simulink model "ThermalConv"  (R2023b)
settings: Solver=FixedStepDiscrete  StartTime=0.0  StopTime=10.0  FixedStep=10e-3  RelTol=1e-3
libraries: AswLib x12
settings Model: DataDictionary=ThermalConv.sldd  Creator=84339  LastModifiedBy=84339
settings OptimizationCC: DefaultParameterBehavior=Inlined  EnhancedBackFolding=on  PassReuseOutputArgsAs=Individual arguments  ZeroExternalMemoryAtStartup=off  ZeroInternalMemoryAtStartup=off  OptimizeBlockOrder=speed  DifferentSizesBufferReuse=on  OptimizationCustomize=off  EfficientTunableParamExpr=on
settings DebuggingCC: ParameterTunabilityLossMsg=error
settings SFSimCC: MATLABDynamicMemAlloc=off
settings RTWCC: Description=Embedded Coder  SystemTargetFile=ert.tlc  EmbeddedCoderDictionary=ASW.sldd  GenCodeOnly=on  TemplateMakefile=ert_default_tmf  DataTypeReplacement=CDataTypesFixedWidth
settings CodeAppCC: ForceParamTrailComments=on  IgnoreCustomStorageClasses=off  OperatorAnnotations=on  SimulinkDataObjDesc=on  SFDataObjDesc=on  InsertBlockDesc=on
settings ERTTargetCC: TargetLangStandard=C99 (ISO)  GenerateSampleERTMain=on  InlinedParameterPlacement=NonHierarchical  ERTCustomFileTemplate=example_file_process.tlc  MaxIdInt64=INT64_MAX  MinIdInt64=INT64_MIN  MaxIdUint64=UINT64_MAX  MaxIdInt32=INT32_MAX  MinIdInt32=INT32_MIN  MaxIdUint32=UINT32_MAX  MaxIdInt16=INT16_MAX  MinIdInt16=INT16_MIN  MaxIdUint16=UINT16_MAX  MaxIdInt8=INT8_MAX  MinIdInt8=INT8_MIN  MaxIdUint8=UINT8_MAX

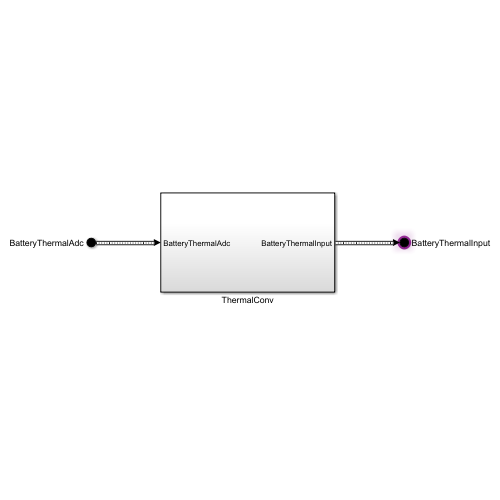
[thumbnail: Simulink's stored preview of the top-level diagram]
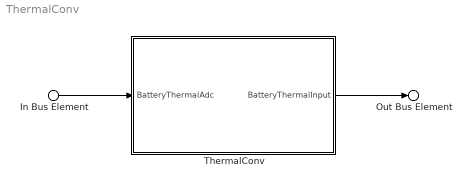
== system ThermalConv ==
  In Bus Element : Inport  PortName=BatteryThermalAdc
  ThermalConv : Subsystem
  Out Bus Element : Outport  PortName=BatteryThermalInput
  wires:
  In Bus Element/1 -> ThermalConv/1(BatteryThermalAdc)
  ThermalConv/1(BatteryThermalInput) -> Out Bus Element/1

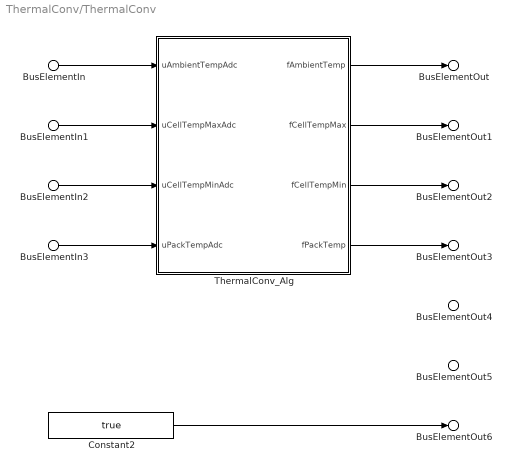
== system ThermalConv/ThermalConv ==
  BusElementIn : Inport  PortName=BatteryThermalAdc  Element=uAmbientTempAdc
  BusElementIn1 : Inport  PortName=BatteryThermalAdc  Element=uCellTempMaxAdc
  BusElementIn3 : Inport  PortName=BatteryThermalAdc  Element=uPackTempAdc
  BusElementIn2 : Inport  PortName=BatteryThermalAdc  Element=uCellTempMinAdc
  Constant2 : Constant  Value=true  OutDataTypeStr=boolean
  ThermalConv_Alg : Subsystem
  BusElementOut1 : Outport  PortName=BatteryThermalInput  Element=fCellTempMax
  BusElementOut2 : Outport  PortName=BatteryThermalInput  Element=fCellTempMin
  BusElementOut3 : Outport  PortName=BatteryThermalInput  Element=fPackTemp
  BusElementOut5 : Outport  PortName=BatteryThermalInput  Element=fChargeCurrent
  BusElementOut : Outport  PortName=BatteryThermalInput  Element=fAmbientTemp
  BusElementOut6 : Outport  PortName=BatteryThermalInput  Element=bSensorValid
  BusElementOut4 : Outport  PortName=BatteryThermalInput  Element=fDischargeCurrent
  wires:
  BusElementIn/1 -> ThermalConv_Alg/1(uAmbientTempAdc)
  BusElementIn1/1 -> ThermalConv_Alg/2(uCellTempMaxAdc)
  BusElementIn2/1 -> ThermalConv_Alg/3(uCellTempMinAdc)
  BusElementIn3/1 -> ThermalConv_Alg/4(uPackTempAdc)
  ThermalConv_Alg/1(fAmbientTemp) -> BusElementOut/1
  ThermalConv_Alg/2(fCellTempMax) -> BusElementOut1/1
  ThermalConv_Alg/3(fCellTempMin) -> BusElementOut2/1
  ThermalConv_Alg/4(fPackTemp) -> BusElementOut3/1
  Constant2/1 -> BusElementOut6/1

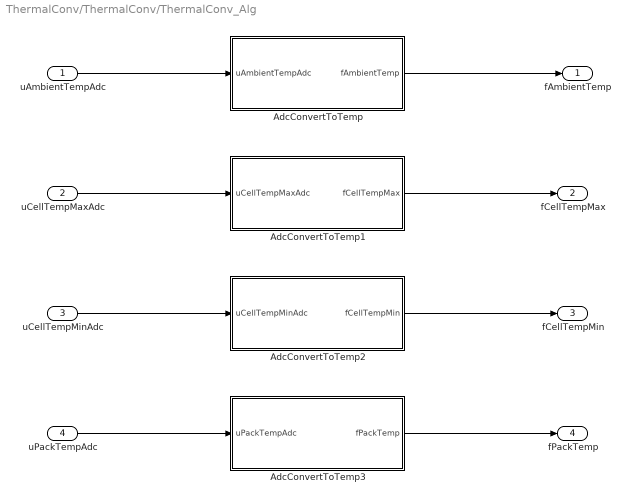
== system ThermalConv/ThermalConv/ThermalConv_Alg ==
  uAmbientTempAdc : Inport
  uCellTempMaxAdc : Inport  Port=2
  uCellTempMinAdc : Inport  Port=3
  uPackTempAdc : Inport  Port=4
  AdcConvertToTemp : Subsystem  TreatAsAtomicUnit=on
      settings: RTWFcnNameOpts=Use subsystem name
  AdcConvertToTemp1 : Subsystem  TreatAsAtomicUnit=on
      settings: RTWFcnNameOpts=Use subsystem name
  AdcConvertToTemp2 : Subsystem  TreatAsAtomicUnit=on
      settings: RTWFcnNameOpts=Use subsystem name
  AdcConvertToTemp3 : Subsystem  TreatAsAtomicUnit=on
      settings: RTWFcnNameOpts=Use subsystem name
  fAmbientTemp : Outport
  fCellTempMax : Outport  Port=2
  fCellTempMin : Outport  Port=3
  fPackTemp : Outport  Port=4
  wires:
  uAmbientTempAdc/1 -> AdcConvertToTemp/1(uAmbientTempAdc)
  AdcConvertToTemp/1(fAmbientTemp) -> fAmbientTemp/1
  uCellTempMaxAdc/1 -> AdcConvertToTemp1/1(uCellTempMaxAdc)
  AdcConvertToTemp1/1(fCellTempMax) -> fCellTempMax/1
  uCellTempMinAdc/1 -> AdcConvertToTemp2/1(uCellTempMinAdc)
  AdcConvertToTemp2/1(fCellTempMin) -> fCellTempMin/1
  AdcConvertToTemp3/1(fPackTemp) -> fPackTemp/1
  uPackTempAdc/1 -> AdcConvertToTemp3/1(uPackTempAdc)

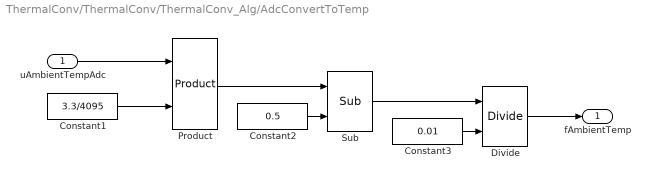
== system ThermalConv/ThermalConv/ThermalConv_Alg/AdcConvertToTemp ==
  uAmbientTempAdc : Inport
  Constant1 : Constant  Value=3.3/4095  OutDataTypeStr=single
  Constant2 : Constant  Value=0.5  OutDataTypeStr=single
  Constant3 : Constant  Value=0.01  OutDataTypeStr=single
  Divide : AswLib/Divide  SystemSampleTime=-1  VariantActivationTime=update diagram  AllowFlexibleInterface=on  Latency=0  AutoFrameSizeCalculation=off
  Product : AswLib/Product  SystemSampleTime=-1  VariantActivationTime=update diagram  AllowFlexibleInterface=on  Latency=0  AutoFrameSizeCalculation=off
  Sub : AswLib/Sub  SystemSampleTime=-1  VariantActivationTime=update diagram  AllowFlexibleInterface=on  Latency=0  AutoFrameSizeCalculation=off
  fAmbientTemp : Outport
  wires:
  Product/1 -> Sub/1
  Divide/1 -> fAmbientTemp/1
  Constant1/1 -> Product/2
  Constant2/1 -> Sub/2
  Sub/1 -> Divide/1
  Constant3/1 -> Divide/2
  uAmbientTempAdc/1 -> Product/1

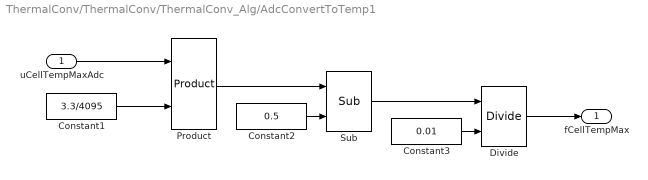
== system ThermalConv/ThermalConv/ThermalConv_Alg/AdcConvertToTemp1 ==
  uCellTempMaxAdc : Inport
  Constant1 : Constant  Value=3.3/4095  OutDataTypeStr=single
  Constant2 : Constant  Value=0.5  OutDataTypeStr=single
  Constant3 : Constant  Value=0.01  OutDataTypeStr=single
  Divide : AswLib/Divide  SystemSampleTime=-1  VariantActivationTime=update diagram  AllowFlexibleInterface=on  Latency=0  AutoFrameSizeCalculation=off
  Product : AswLib/Product  SystemSampleTime=-1  VariantActivationTime=update diagram  AllowFlexibleInterface=on  Latency=0  AutoFrameSizeCalculation=off
  Sub : AswLib/Sub  SystemSampleTime=-1  VariantActivationTime=update diagram  AllowFlexibleInterface=on  Latency=0  AutoFrameSizeCalculation=off
  fCellTempMax : Outport
  wires:
  Product/1 -> Sub/1
  Divide/1 -> fCellTempMax/1
  Constant1/1 -> Product/2
  Constant2/1 -> Sub/2
  Sub/1 -> Divide/1
  Constant3/1 -> Divide/2
  uCellTempMaxAdc/1 -> Product/1

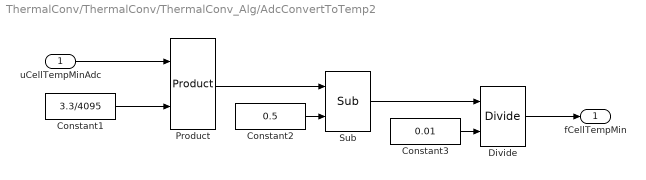
== system ThermalConv/ThermalConv/ThermalConv_Alg/AdcConvertToTemp2 ==
  uCellTempMinAdc : Inport
  Constant1 : Constant  Value=3.3/4095  OutDataTypeStr=single
  Constant2 : Constant  Value=0.5  OutDataTypeStr=single
  Constant3 : Constant  Value=0.01  OutDataTypeStr=single
  Divide : AswLib/Divide  SystemSampleTime=-1  VariantActivationTime=update diagram  AllowFlexibleInterface=on  Latency=0  AutoFrameSizeCalculation=off
  Product : AswLib/Product  SystemSampleTime=-1  VariantActivationTime=update diagram  AllowFlexibleInterface=on  Latency=0  AutoFrameSizeCalculation=off
  Sub : AswLib/Sub  SystemSampleTime=-1  VariantActivationTime=update diagram  AllowFlexibleInterface=on  Latency=0  AutoFrameSizeCalculation=off
  fCellTempMin : Outport
  wires:
  Product/1 -> Sub/1
  Divide/1 -> fCellTempMin/1
  Constant1/1 -> Product/2
  Constant2/1 -> Sub/2
  Sub/1 -> Divide/1
  Constant3/1 -> Divide/2
  uCellTempMinAdc/1 -> Product/1

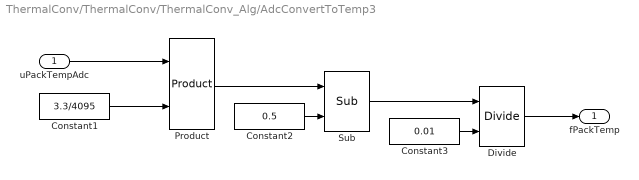
== system ThermalConv/ThermalConv/ThermalConv_Alg/AdcConvertToTemp3 ==
  uPackTempAdc : Inport
  Constant1 : Constant  Value=3.3/4095  OutDataTypeStr=single
  Constant2 : Constant  Value=0.5  OutDataTypeStr=single
  Constant3 : Constant  Value=0.01  OutDataTypeStr=single
  Divide : AswLib/Divide  SystemSampleTime=-1  VariantActivationTime=update diagram  AllowFlexibleInterface=on  Latency=0  AutoFrameSizeCalculation=off
  Product : AswLib/Product  SystemSampleTime=-1  VariantActivationTime=update diagram  AllowFlexibleInterface=on  Latency=0  AutoFrameSizeCalculation=off
  Sub : AswLib/Sub  SystemSampleTime=-1  VariantActivationTime=update diagram  AllowFlexibleInterface=on  Latency=0  AutoFrameSizeCalculation=off
  fPackTemp : Outport
  wires:
  Product/1 -> Sub/1
  Divide/1 -> fPackTemp/1
  Constant1/1 -> Product/2
  Constant2/1 -> Sub/2
  Sub/1 -> Divide/1
  Constant3/1 -> Divide/2
  uPackTempAdc/1 -> Product/1
